simulink model "L8"  (R2015a)
settings: Solver=ode45  StartTime=0.0  StopTime=10.0  RelTol=1e-3
libraries: commdigbbndpm3 x2, commchan3 x1, commsink2 x1, commrandsrc2 x1
settings Model: Creator=User  LastModifiedBy=User

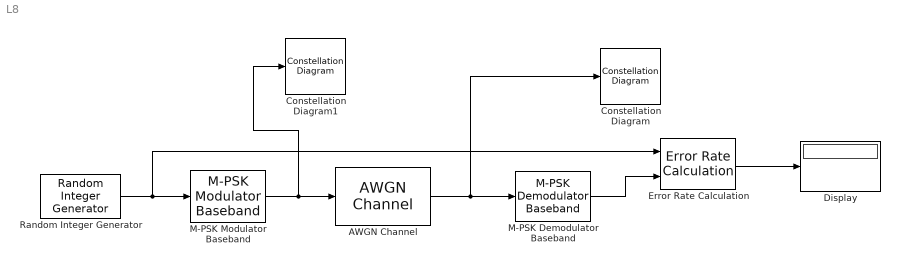
== system L8 ==
  AWGN Channel : commchan3/AWGN Channel  InputProcessing=Columns as channels (frame based)  seed=67  noiseMode="Signal to noise ratio  (Eb/No)"  EbNodB=15  EsNodB=10  SNRdB=10  bitsPerSym=4  Ps=1  Tsym=2e-6  variance=1
  Constellation Diagram : ConstellationDiagram
  Constellation Diagram1 : ConstellationDiagram
  Display : Display
  Error Rate Calculation : commsink2/Error Rate Calculation  N=0  st_delay=0  cp_mode=Entire frame  subframe=[]  PMode=Port  WsName=ErrorVec  RsMode2=off  stop=off  numErr=100  maxBits=1e6
  M-PSK Demodulator Baseband : commdigbbndpm3/M-PSK Demodulator Baseband  M=256  Ph=pi/8  Dec=Gray  Mapping=[0:7]  OutType=Integer  DecType=Hard decision  VarSource=Dialog  Variance=1  outDtype1=Inherit via internal rule  outDtype2=Inherit via internal rule  derotateFactorWordLen=16
  M-PSK Modulator Baseband : commdigbbndpm3/M-PSK Modulator Baseband  M=256  InType=Integer  Enc=Gray  Mapping=[0:7]  Ph=pi/8  outDtype=double  outWordLen=16  outUDDataType=sfix(16)  outFracLenMode=Best precision  outFracLen=15
  Random Integer Generator : commrandsrc2/Random Integer Generator  mul=256  seed=37  Ts=2e-6  frameBased=off  sampPerFrame=1  orient=off  outDataType=double
  wires:
  Random Integer Generator/1 -> M-PSK Modulator Baseband/1, Error Rate Calculation/1
  M-PSK Modulator Baseband/1 -> Constellation Diagram1/1, AWGN Channel/1
  M-PSK Demodulator Baseband/1 -> Error Rate Calculation/2
  AWGN Channel/1 -> M-PSK Demodulator Baseband/1, Constellation Diagram/1
  Error Rate Calculation/1 -> Display/1
